simulink model "color_separate"  (R2015a)
settings: Solver=ode45  StartTime=0.0  StopTime=inf  RelTol=1e-3
undefined symbols (not defined in the file or in its folder): gray, IsPositionTracked, IsSkeletonTracked, JointDepthIndices, JointImageIndices, JointTrackingState, JointWorldCoordinates, none, PositionDepthIndices, PositionImageIndices, PositionWorldCoordinates, Rec, SDTV, SegmentationData, SkeletonTrackingID, videoinput
libraries: simulink x3, visionsinks x2, visionconversions x1, imaqlib x1
settings Model: Creator=Grisha  LastModifiedBy=Grisha

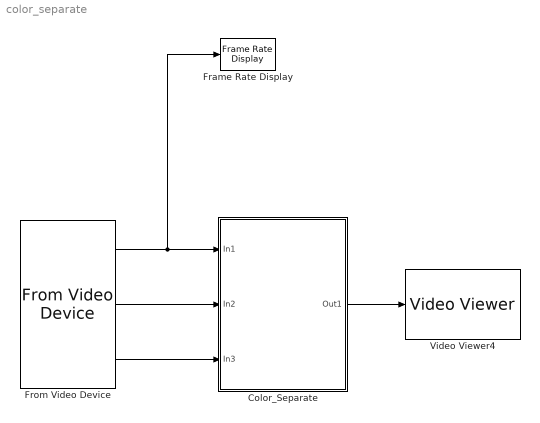
== system color_separate ==
  Color_Separate : Subsystem
  Frame Rate Display : visionsinks/Frame Rate Display  UpdateRate=10
  From Video Device : imaqlib/From Video Device  DeviceMenu=winvideo 1 (QuickCam Orbit/Sphere AF)  Device=winvideo 1 (QuickCam Orbit/Sphere AF)  ObjConstructor=videoinput('winvideo', 1)  VideoFormatMenu=RGB24_1280x800  VideoFormat=RGB24_1280x800  VideoSource=input1  ROIPosition=[0 0 800 1280]  EnableHWTrigger=off  TriggerConfiguration=none/none  SampleTime=1/30  OutputPortsMode=Separate color signals  DataType=double  CanDoHWTrigger=no  ReturnedColorSpace=rgb  BlockHandle=1930.0004  ROIWidth=1280  ROIHeight=800  ROIColumn=0  ROIRow=0  EngXMLPath=C:\Program Files\MATLAB\MATLAB Production Server\R2015a\toolbox\imaq\imaq\private  DevXMLPath=C:\MATLAB\SupportPackages\R2015a\osgenericvideointerface\toolbox\imaq\supportpackages\genericvideo\adaptor\win64  EngLibPath=C:\Program Files\MATLAB\MATLAB Production Server\R2015a\toolbox\imaq\imaqblks\imaqmex\win64  ColorSpace=rgb  BayerSensorAlignment=grbg  AllMetadata=IsPositionTracked;IsSkeletonTracked;JointDepthIndices;JointImageIndices;JointTrackingState;JointWorldCoordinates;PositionDepthIndices;PositionImageIndices;PositionWorldCoordinates;SegmentationData;SkeletonTrackingID
  Video Viewer4 : visionsinks/Video Viewer  inputType=Obsolete7b  imagePorts=One multidimensional signal  useColorMap=off  colormapValue=gray(256)  specRange=off  minInputVal=0  maxInputVal=255  FigPos=[93 862 804 572]  AxisZoom=on  trueSizedOnce=off  OpenAtMdlStart=on  DefaultConfigurationName=vipscopes.VideoViewerScopeCfg
  wires:
  From Video Device/1 -> Color_Separate/1(In1), Frame Rate Display/1
  Color_Separate/1(Out1) -> Video Viewer4/1
  From Video Device/2 -> Color_Separate/2(In2)
  From Video Device/3 -> Color_Separate/3(In3)

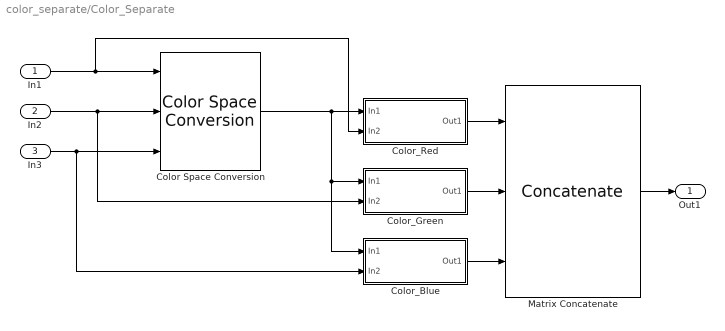
== system color_separate/Color_Separate ==
  In1 : Inport
  In2 : Inport  Port=2
  In3 : Inport  Port=3
  Color Space Conversion : visionconversions/Color Space  Conversion  conversion=Obsolete  conversionActive=R'G'B' to intensity  wp_str=D65  rec=Rec. 601 (SDTV)  sys=1125/60/2:1  imagePorts=Separate color signals
  Color_Blue : Subsystem
  Color_Green : Subsystem
  Color_Red : Subsystem
  Matrix Concatenate : Concatenate  NumInputs=3  Mode=Multidimensional array  ConcatenateDimension=3
  Out1 : Outport
  wires:
  Color_Red/1(Out1) -> Matrix Concatenate/1
  Color_Blue/1(Out1) -> Matrix Concatenate/3
  Color_Green/1(Out1) -> Matrix Concatenate/2
  Matrix Concatenate/1 -> Out1/1
  Color Space Conversion/1 -> Color_Green/1(In1), Color_Blue/1(In1), Color_Red/1(In1)
  In2/1 -> Color Space Conversion/2, Color_Green/2(In2)
  In3/1 -> Color_Blue/2(In2), Color Space Conversion/3
  In1/1 -> Color_Red/2(In2), Color Space Conversion/1

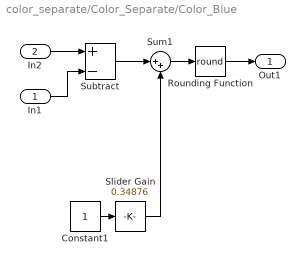
== system color_separate/Color_Separate/Color_Blue ==
  In1 : Inport
  In2 : Inport  Port=2
  Constant1 : Constant
  Rounding Function : Rounding  Operator=round
  Slider Gain : simulink/Math Operations/Slider Gain  low=0  gain=0.34876  high=1
  Subtract : Sum  Inputs=+-
  Sum1 : Sum  Inputs=|++  RndMeth=Round
  Out1 : Outport
  wires:
  Subtract/1 -> Sum1/1
  Sum1/1 -> Rounding Function/1
  In2/1 -> Subtract/1
  In1/1 -> Subtract/2
  Rounding Function/1 -> Out1/1
  Constant1/1 -> Slider Gain/1
  Slider Gain/1 -> Sum1/2

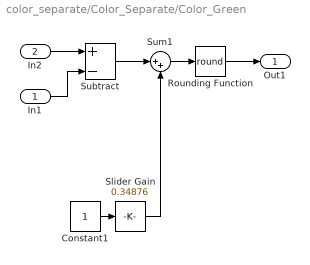
== system color_separate/Color_Separate/Color_Green ==
  In1 : Inport
  In2 : Inport  Port=2
  Constant1 : Constant
  Rounding Function : Rounding  Operator=round
  Slider Gain : simulink/Math Operations/Slider Gain  low=0  gain=0.34876  high=1
  Subtract : Sum  Inputs=+-
  Sum1 : Sum  Inputs=|++  RndMeth=Round
  Out1 : Outport
  wires:
  Subtract/1 -> Sum1/1
  Sum1/1 -> Rounding Function/1
  In2/1 -> Subtract/1
  In1/1 -> Subtract/2
  Rounding Function/1 -> Out1/1
  Constant1/1 -> Slider Gain/1
  Slider Gain/1 -> Sum1/2

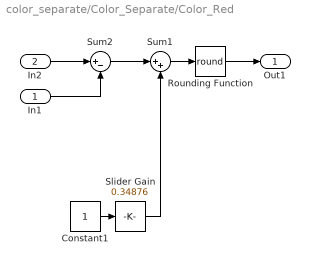
== system color_separate/Color_Separate/Color_Red ==
  In1 : Inport
  In2 : Inport  Port=2
  Constant1 : Constant
  Rounding Function : Rounding  Operator=round
  Slider Gain : simulink/Math Operations/Slider Gain  low=0  gain=0.34876  high=1
  Sum1 : Sum  Inputs=|++  RndMeth=Round
  Sum2 : Sum  Inputs=|+-  RndMeth=Round
  Out1 : Outport
  wires:
  Sum2/1 -> Sum1/1
  Sum1/1 -> Rounding Function/1
  Rounding Function/1 -> Out1/1
  Constant1/1 -> Slider Gain/1
  In2/1 -> Sum2/1
  In1/1 -> Sum2/2
  Slider Gain/1 -> Sum1/2
